simulink model "ecos_simulink_demo_R2016b"  (R2016b)
settings: Solver=VariableStepAuto  StartTime=0.0  StopTime=1  RelTol=1e-3
undefined symbols (not defined in the file): Air_size, Ajc_size, Apr_size, b_size, c_size, Gir_size, Gjc_size, Gpr_size, h_size, q_size
settings Model: Creator=danylo  LastModifiedBy=Taylor
settings SFSimCC: SimUseLocalCustomCode=on
settings RTWCC: RTWUseLocalCustomCode=on

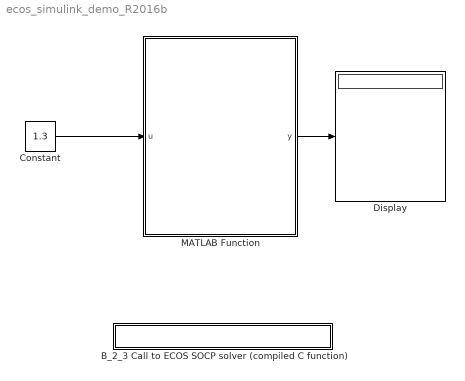
== system ecos_simulink_demo_R2016b ==
  B_2_3 Call to ECOS SOCP solver (compiled C function) : Subsystem  TreatAsAtomicUnit=on
  Constant : Constant  Value=1.3
  Display : Display
  MATLAB Function : MATLAB Function  TreatAsAtomicUnit=on
  wires:
  MATLAB Function/1(y) -> Display/1
  Constant/1 -> MATLAB Function/1(u)

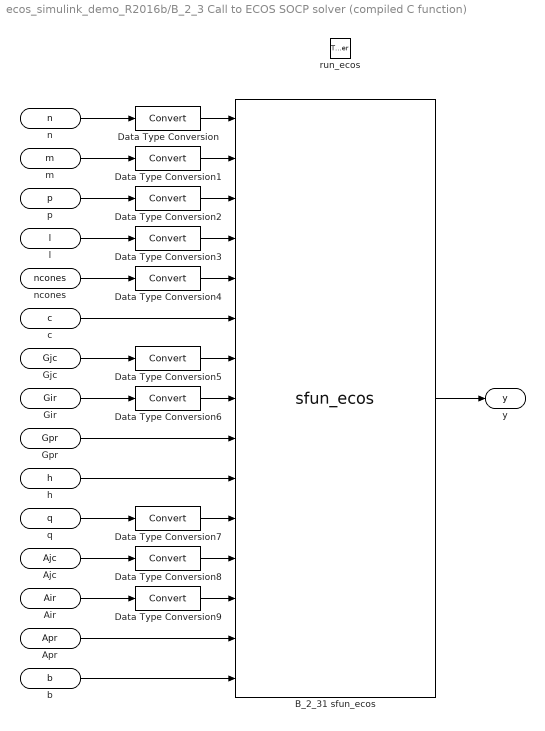
== system ecos_simulink_demo_R2016b/B_2_3 Call to ECOS SOCP solver (compiled C function) ==
  run_ecos : TriggerPort  TriggerType=function-call  IsSimulinkFunction=on  FunctionName=run_ecos  VariantControl=(inherit)
  B_2_31 sfun_ecos : S-Function  FunctionName=sfun_ecos  SFunctionDeploymentMode=off  EnableBusSupport=off  mask(Legacy Function){}
      mask help:
      | This block allows you to call the legacy functions specified by the following Legacy Code Tool definition:
      | def.SFunctionName = 'sfun_ecos';
      | def.OutputFcnSpec = 'solve_simple_optimization(int32 p1,int32 p2,int32 p3,int32 p4,int32 p5,double p6[18],int32 p7[19],int32 p8[57],double u1[57],double u2[38],int32 p9[6],int32 p10[19],int32 p11[16],double u3[16],double u4[6],solution y1[1])';
      | def.HeaderFiles = {'ecos.h', 'matlab_header.h'};
      | def.SourceFiles = {'main.c', 'cone.c', 'ctrlc.c', 'ecos.c', 'equil.c', 'expcone.c', 'kkt.c', 'preproc.c', 'spla.c', 'splamm.c', 'timer.c', 'wright_omega.c', 'ldl.c', 'amd_1.c', 'amd_2.c', 'amd_aat.c', 'amd_control.c', 'amd_defaults.c', 'amd_dump.c', 'amd_global.c', 'amd_info.c', 'amd_order.c', 'amd_post_tree.c', 'amd_postorder.c', 'amd_preprocess.c', 'amd_valid.c'};
      | def.IncPaths = {'./ecos/include', './ecos/external/ldl/include', './ecos/external/amd/include', './ecos/external/SuiteSparse_config'};
      | def.SrcPaths = {'./ecos/src', './ecos/external/ldl/src', './ecos/external/amd/src'};
      mask Help: <p>This block was generated automatically by the Legacy Code Tool. For detailed help on this tool, call<a href="matlab:legacy_code('help')"> legacy_code('help')</a>.</p>
      mask DialogControl DescGroupVar Prompt: Convex optimization
      mask DialogControl DescTextVar Prompt: <b>Mathematical description</b><br><br> Computes optimal power limit trajectory by solving a minimum-time bounded-energy problem via convex optimization. Formulation: <br> <br> min c'*z<br>subject to<br>A*z=b<br>G*z&lt;=_K h <br> <br> Where &lt;=_K denotes a generalized inequality with respect to the cone K, i.e. the vector h-G*z belongs to the cone K. The cone K may be an n-dimensional positive orthant (R_+^n, which simply means G*z &lt;=h is the usual inequality) or a second-order Q^n defined as: <br> <br> Q^n = {(t(z),x(z)) in R x R^{n-1} | t(z) &lt;= ||x(z)||_2} <br> <br> For the latter case, h-G*z defines then the (t,x) in R^n vector. The case of exponential cones, which ECOS can handle, does not appear in the car energy optimization problem and thus is not considered here.<br><br> <b>ECOS C API</b><br><br> n : Number of primal variables<br> m : Number of generalized inequality constraints, i.e. dimension 1 of matrix G and length of vector h<br> p : Number of equality constraints, i.e. dimension 1 of matrix A and length of vector b<br> l : Dimension of the positive orthan R_+^l (number of usual inequality constraints)<br> ncones : Number of second-order cones<br> q : Array of length ncones; q[i] defines the dimension of the cone i<br> Gpr, Gjc, Gir : Arrays of matrix G in column compressed storage (CCS)<br> Apr, Ajc, Air : Arrays of matrix A in column compressed storage (CCS)<br> c : Array of length n (cost)<br> h : Array of length m (RHS of generalized inequality constraints)<br> b : Array of length p (RHS of equality constraints)<br>
      mask Display:
      | %%% Input port labels
      | port_label('input',1,'n');
      | port_label('input',2,'m');
      | port_label('input',3,'p');
      | port_label('input',4,'l');
      | port_label('input',5,'ncones');
      | port_label('input',6,'c');
      | port_label('input',7,'Gjc');
      | port_label('input',8,'Gir');
      | port_label('input',9,'Gpr');
      | port_label('input',10,'h');
      | port_label('input',11,'q');
      | port_label('input',12,'Ajc');
      | port_label('input',13,'Air');
      | port_label('input',14,'Apr');
      | port_label('input',15,'b');
      | port_label('input',16,'Ns');
      | port_label('input',17,'Nu');
      | %%% Outputs port labels
      | port_label('output',1,'optimal_solution');
  Data Type Conversion{,1..9} (10 alike) : DataTypeConversion
  n : ArgIn  DisableCoverage=on  ArgumentName=n
  m : ArgIn  DisableCoverage=on  Port=2  ArgumentName=m
  p : ArgIn  DisableCoverage=on  Port=3  ArgumentName=p
  l : ArgIn  DisableCoverage=on  Port=4  ArgumentName=l
  ncones : ArgIn  DisableCoverage=on  Port=5  ArgumentName=ncones
  c : ArgIn  DisableCoverage=on  Port=6  PortDimensions=c_size  ArgumentName=c
  Gjc : ArgIn  DisableCoverage=on  Port=7  PortDimensions=Gjc_size  ArgumentName=Gjc
  Gir : ArgIn  DisableCoverage=on  Port=8  PortDimensions=Gir_size  ArgumentName=Gir
  Gpr : ArgIn  DisableCoverage=on  Port=9  PortDimensions=Gpr_size  ArgumentName=Gpr
  h : ArgIn  DisableCoverage=on  Port=10  PortDimensions=h_size  ArgumentName=h
  q : ArgIn  DisableCoverage=on  Port=11  PortDimensions=q_size  ArgumentName=q
  Ajc : ArgIn  DisableCoverage=on  Port=12  PortDimensions=Ajc_size  ArgumentName=Ajc
  Air : ArgIn  DisableCoverage=on  Port=13  PortDimensions=Air_size  ArgumentName=Air
  Apr : ArgIn  DisableCoverage=on  Port=14  PortDimensions=Apr_size  ArgumentName=Apr
  b : ArgIn  DisableCoverage=on  Port=15  PortDimensions=b_size  ArgumentName=b
  y : ArgOut  DisableCoverage=on  PortDimensions=y_size  ArgumentName=y
  wires:
  B_2_31 sfun_ecos/1 -> y/1
  n/1 -> Data Type Conversion/1
  m/1 -> Data Type Conversion1/1
  p/1 -> Data Type Conversion2/1
  l/1 -> Data Type Conversion3/1
  ncones/1 -> Data Type Conversion4/1
  Ajc/1 -> Data Type Conversion8/1
  Air/1 -> Data Type Conversion9/1
  Apr/1 -> B_2_31 sfun_ecos/14
  b/1 -> B_2_31 sfun_ecos/15
  c/1 -> B_2_31 sfun_ecos/6
  Gjc/1 -> Data Type Conversion5/1
  Gir/1 -> Data Type Conversion6/1
  Gpr/1 -> B_2_31 sfun_ecos/9
  h/1 -> B_2_31 sfun_ecos/10
  q/1 -> Data Type Conversion7/1
  Data Type Conversion/1 -> B_2_31 sfun_ecos/1
  Data Type Conversion1/1 -> B_2_31 sfun_ecos/2
  Data Type Conversion2/1 -> B_2_31 sfun_ecos/3
  Data Type Conversion3/1 -> B_2_31 sfun_ecos/4
  Data Type Conversion4/1 -> B_2_31 sfun_ecos/5
  Data Type Conversion5/1 -> B_2_31 sfun_ecos/7
  Data Type Conversion6/1 -> B_2_31 sfun_ecos/8
  Data Type Conversion7/1 -> B_2_31 sfun_ecos/11
  Data Type Conversion8/1 -> B_2_31 sfun_ecos/12
  Data Type Conversion9/1 -> B_2_31 sfun_ecos/13

== matlab function ecos_simulink_demo_R2016b/MATLAB Function ==
  data: u input; y output; c_size parameter; Air_size parameter; Ajc_size parameter; Apr_size parameter; b_size parameter; Gir_size parameter; Gjc_size parameter; Gpr_size parameter; h_size parameter; q_size parameter
function y = optimize(u,c_size, Air_size, Ajc_size, Apr_size, b_size, Gir_size, Gjc_size, Gpr_size, h_size, q_size)
% Data
n = 2;
m = 5;
p = 1;
l = 2;
ncones = 1;
e = 0;
c = [0;1];
G = [1 -1;-1 -1;0 0;-1 0;0 -1];
h = [0;-2;2;0;0];
A = [1 0];
b = u;
q = [3];

[Air,Ajc,Apr] = convert_to_CCS(A);
[Gir,Gjc,Gpr] = convert_to_CCS(G);

% CHANGE THINGS ABOVE

% Call to ECOS
y = run_ecos(n,m,p,l,ncones,c(1:c_size),Gjc(1:Gjc_size),Gir(1:Gir_size),Gpr(1:Gpr_size),...
             h(1:h_size),q(1:q_size),Ajc(1:Ajc_size),Air(1:Air_size),Apr(1:Apr_size),b(1:b_size));
end

function [Mir,Mjc,Mpr] = convert_to_CCS(Mf)
[Mir,~,Mpr] = find(Mf);
Mir = Mir-1; % zero-based row indexing
Mjc = zeros(size(Mf,2)+1,1);
for col = 2:size(Mf,2)
    Mjc(col) = Mjc(col-1)+nnz(Mf(:,col-1));
end
Mjc(end) = length(find(Mf~=0));
end
